simulink model "TX_TUNE_DIGITAL"  (R2024a)
settings: Solver=VariableStepAuto  StartTime=0.0  StopTime=1e-3  FixedStep=1e-9  RelTol=1e-3
values from neighbouring files (symbols this model uses):
  cnt_n_bits = 9    [TX_PM_MODEL_Setup.m]
  Cs = 12.5e-12    (= 1.25e-11)    [Oscillator_Setup.m]
  deltaVOSC = 0.5    [Oscillator_Setup.m]
  I0 = 100e-6    (= 0.0001)    [Oscillator_Setup.m]
  R = 0.2    [TX_PM_MODEL_Setup.m]
  Rf = 1e9    (= 1000000000)    [Oscillator_Setup.m]
  VDD = 5    [Oscillator_Setup.m]    (also in TX_PM_MODEL_Setup.m = 10)
  Vh = VDD - deltaVOSC    (= 4.5)    [Oscillator_Setup.m]
  Vl = deltaVOSC    (= 0.5)    [Oscillator_Setup.m]
undefined symbols (not defined in the file or in its folder): VDD_DRIVE
libraries: fl_lib x12, nesl_utility x7, MyLib x3, dspsigops x3, ee_lib x1, spsTriangleGeneratorLib x1
settings Model: Creator=cian.odonnell  LastModifiedBy=ciano
settings SolverCC: EnableFixedStepZeroCrossing=on

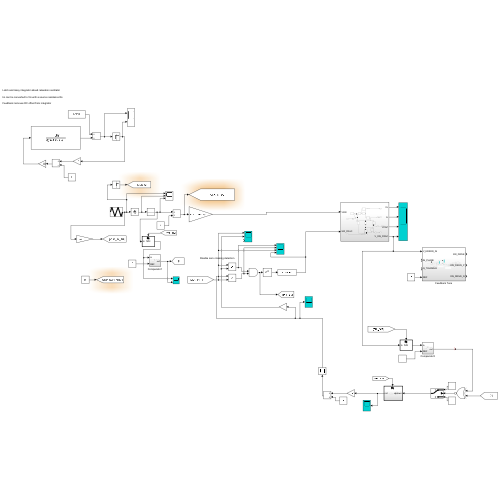
[thumbnail: Simulink's stored preview of the top-level diagram]
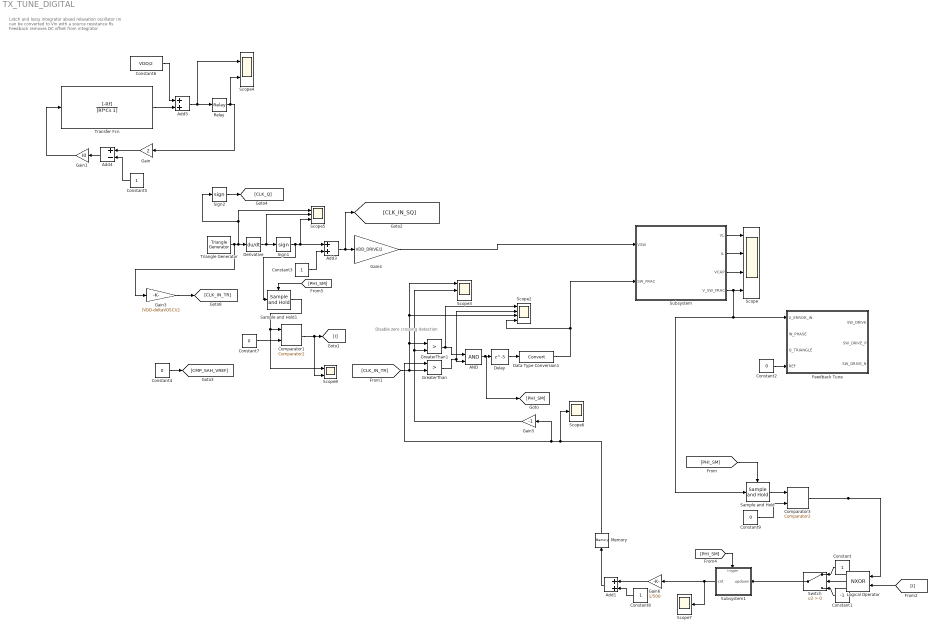
== system TX_TUNE_DIGITAL ==
  note: Latch and lossy integrator absed relaxation oscillator
      |
      | Iin can be converted to Vin with a source resistance Rs
      |
      | Feedback removes DC offset from integrator
  note: Disable zero crossing detection
  AND : Logic  IconShape=distinctive  AllPortsSameDT=off  OutDataTypeStr=boolean
  Add1 : Sum
  Add3 : Sum
  Add4 : Sum  Inputs=+-
  Add5 : Sum
  Comparator1 : MyLib/Comparator2  SystemSampleTime=-1  VariantActivationTime=update diagram  AllowFlexibleInterface=on  Latency=0  AutoFrameSizeCalculation=off
  Comparator3 : MyLib/Comparator2  SystemSampleTime=-1  VariantActivationTime=update diagram  AllowFlexibleInterface=on  Latency=0  AutoFrameSizeCalculation=off
  Constant{,3,5,8} (4 alike) : Constant
  Constant1 : Constant  Value=-1
  Constant{2,4,7,9} (4 alike) : Constant  Value=0
  Constant6 : Constant  Value=VDD/2
  Data Type Conversion1 : DataTypeConversion  SaturateOnIntegerOverflow=off  RndMeth=Floor
  Delay : Delay  DelayLength=5  SampleTime=1e-9
  Derivative : Derivative
  Feedback Tune : Subsystem
  Gain : Gain  Gain=2
  Gain1 : Gain  Gain=I0
  Gain3 : Gain  Gain=(VDD-deltaVOSC)/2
  Gain4 : Gain  Gain=VDD_DRIVE/2
  Gain5 : Gain  Gain=-1
  Gain6 : Gain  Gain=1/500
  GreaterThan : RelationalOperator  Operator=>  OutDataTypeStr=boolean  ZeroCross=off  RndMeth=Simplest  InputSameDT=off
  GreaterThan1 : RelationalOperator  Operator=>  OutDataTypeStr=boolean  ZeroCross=off  RndMeth=Simplest  InputSameDT=off
  Logical Operator : Logic  Operator=NXOR  IconShape=distinctive  AllPortsSameDT=off  OutDataTypeStr=boolean
  Memory : Memory
  Relay : Relay  OnSwitchValue=Vh  OffSwitchValue=Vl
  Sample and Hold : dspsigops/Sample and Hold  trig=Either edge  initCond=0  latchinput=off
  Sample and Hold1 : dspsigops/Sample and Hold  trig=Either edge  initCond=0  latchinput=off
  Scope : Scope  NumInputPorts=4
  Scope2 : Scope  NumInputPorts=4
  Scope3 : Scope  NumInputPorts=3
  Scope4 : Scope  NumInputPorts=2
  Scope5 : Scope  NumInputPorts=3
  Scope6 : Scope
  Scope7 : Scope
  Scope8 : Scope  NumInputPorts=2
  Sign1 : Signum
  Sign2 : Signum
  Subsystem : Subsystem
  Subsystem1 : Subsystem
  Switch : Switch  Criteria=u2 > Threshold  SaturateOnIntegerOverflow=off  InputSameDT=off
  Transfer Fcn : TransferFcn  Numerator=[-Rf]  Denominator=[Rf*Cs 1]
  Triangle Generator : spsTriangleGeneratorLib/Triangle Generator  Freq=fin  Phase=90  Ts=0
  wires:
  GreaterThan/1 -> Scope2/2, AND/2
  Add5/1 -> Scope4/1, Relay/1
  Transfer Fcn/1 -> Add5/2
  Gain1/1 -> Transfer Fcn/1
  Add4/1 -> Gain1/1
  Gain/1 -> Add4/1
  Constant5/1 -> Add4/2
  Constant6/1 -> Add5/1
  Relay/1 -> Gain/1, Scope4/2
  Gain3/1 -> [CLK_IN_TR]
  Triangle Generator/1 -> Sign2/1, Scope5/1, Derivative/1, Gain3/1
  Derivative/1 -> Sign1/1, Scope5/2
  Sign1/1 -> Sample and Hold1/1, Add3/1, Scope5/3
  Constant3/1 -> Add3/2
  Add3/1 -> [CLK_IN_SQ], Gain4/1
  [CLK_IN_TR] -> GreaterThan/2, GreaterThan1/1, Scope3/1, Scope2/3
  Gain5/1 -> GreaterThan1/2, Scope3/2
  GreaterThan1/1 -> Scope2/1, AND/1
  Data Type Conversion1/1 -> Scope2/4, Subsystem/2(SW_FRAC)
  AND/1 -> [PHI_SM], Delay/1
  Delay/1 -> Data Type Conversion1/1
  [I] -> Logical Operator/2
  Gain4/1 -> Subsystem/1(VSW)
  Subsystem/1(VL) -> Scope/1
  Subsystem/2(IL) -> Scope/2
  Subsystem/3(VCAP) -> Scope/3
  Comparator1/1 -> Scope8/2, [I]
  Constant4/1 -> [CMP_SAH_VREF]
  Constant7/1 -> Comparator1/2
  Sign2/1 -> [CLK_Q]
  Add1/1 -> Memory/1
  [PHI_SM] -> Subsystem1/Trigger
  Subsystem1/1(cnt) -> Gain6/1, Scope7/1
  Switch/1 -> Subsystem1/1(updown)
  Sample and Hold1/1 -> Comparator1/1, Scope8/1
  [PHI_SM] -> Sample and Hold1/Trigger
  Logical Operator/1 -> Switch/2
  Constant/1 -> Switch/1
  Constant1/1 -> Switch/3
  Gain6/1 -> Add1/1
  Constant8/1 -> Add1/2
  Memory/1 -> Scope6/1, GreaterThan/1, Gain5/1
  Constant2/1 -> Feedback Tune/4(REF)
  Comparator3/1 -> Logical Operator/1
  Sample and Hold/1 -> Comparator3/1
  Subsystem/4(V_SW_FRAC) -> Sample and Hold/1, Feedback Tune/1(V_ERROR_IN), Scope/4
  Constant9/1 -> Comparator3/2
  [PHI_SM] -> Sample and Hold/Trigger

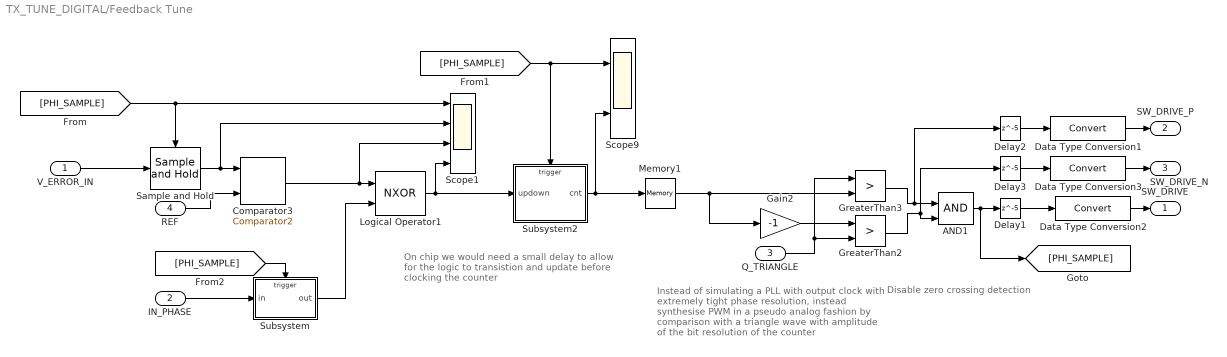
== system TX_TUNE_DIGITAL/Feedback Tune ==
  note: On chip we would need a small delay to allow for the logic to transistion and update before clocking the counter
  note: Disable zero crossing detection
  note: Instead of simulating a PLL with output clock with extremely tight phase resolution, instead synthesise PWM in a pseudo analog fashion by comparison with a triangle wave with amplitude of the bit resolution of the counter
  V_ERROR_IN : Inport
  IN_PHASE : Inport  Port=2
  Q_TRIANGLE : Inport  Port=3
  REF : Inport  Port=4
  AND1 : Logic  IconShape=distinctive  AllPortsSameDT=off  OutDataTypeStr=boolean
  Comparator3 : MyLib/Comparator2  SystemSampleTime=-1  VariantActivationTime=update diagram  AllowFlexibleInterface=on  Latency=0  AutoFrameSizeCalculation=off
  Data Type Conversion1 : DataTypeConversion  SaturateOnIntegerOverflow=off  RndMeth=Floor
  Data Type Conversion2 : DataTypeConversion  SaturateOnIntegerOverflow=off  RndMeth=Floor
  Data Type Conversion3 : DataTypeConversion  SaturateOnIntegerOverflow=off  RndMeth=Floor
  Delay1 : Delay  DelayLength=5  SampleTime=1e-9
  Delay2 : Delay  DelayLength=5  SampleTime=1e-9
  Delay3 : Delay  DelayLength=5  SampleTime=1e-9
  Gain2 : Gain  Gain=-1
  GreaterThan2 : RelationalOperator  Operator=>  OutDataTypeStr=boolean  ZeroCross=off  RndMeth=Simplest  InputSameDT=off
  GreaterThan3 : RelationalOperator  Operator=>  OutDataTypeStr=boolean  ZeroCross=off  RndMeth=Simplest  InputSameDT=off
  Logical Operator1 : Logic  Operator=NXOR  IconShape=distinctive  AllPortsSameDT=off  OutDataTypeStr=boolean
  Memory1 : Memory
  Sample and Hold : dspsigops/Sample and Hold  trig=Either edge  initCond=0  latchinput=off
  Scope1 : Scope  NumInputPorts=4
  Scope9 : Scope  NumInputPorts=2
  Subsystem : Subsystem
  Subsystem2 : Subsystem
  SW_DRIVE : Outport
  SW_DRIVE_P : Outport  Port=2
  SW_DRIVE_N : Outport  Port=3
  wires:
  [PHI_SAMPLE] -> Sample and Hold/Trigger, Scope1/1
  Gain2/1 -> GreaterThan2/1
  Subsystem2/1(cnt) -> Memory1/1, Scope9/2
  Delay1/1 -> Data Type Conversion2/1
  Sample and Hold/1 -> Scope1/2, Comparator3/1
  Logical Operator1/1 -> Subsystem2/1(updown), Scope1/4
  Comparator3/1 -> Scope1/3, Logical Operator1/1
  Memory1/1 -> Gain2/1, GreaterThan3/2
  Q_TRIANGLE/1 -> GreaterThan2/2, GreaterThan3/1
  [PHI_SAMPLE] -> Subsystem2/Trigger, Scope9/1
  GreaterThan3/1 -> Delay2/1, AND1/1
  AND1/1 -> [PHI_SAMPLE], Delay1/1
  GreaterThan2/1 -> Delay3/1, AND1/2
  Data Type Conversion2/1 -> SW_DRIVE/1
  V_ERROR_IN/1 -> Sample and Hold/1
  REF/1 -> Comparator3/2
  IN_PHASE/1 -> Subsystem/1(in)
  Subsystem/1(out) -> Logical Operator1/2
  [PHI_SAMPLE] -> Subsystem/Trigger
  Delay2/1 -> Data Type Conversion1/1
  Delay3/1 -> Data Type Conversion3/1
  Data Type Conversion1/1 -> SW_DRIVE_P/1
  Data Type Conversion3/1 -> SW_DRIVE_N/1

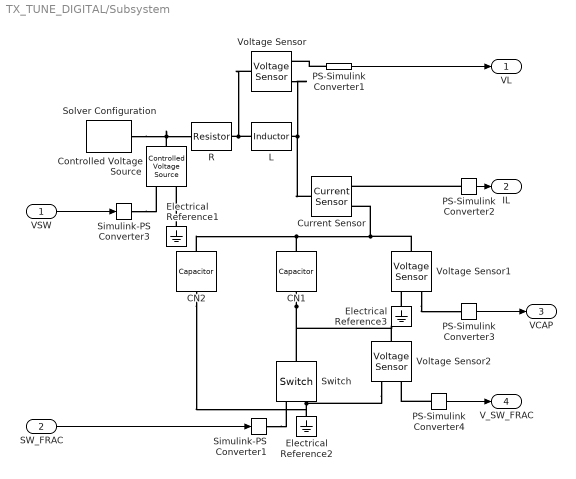
== system TX_TUNE_DIGITAL/Subsystem ==
  VSW : Inport
  SW_FRAC : Inport  Port=2
  CN1 : fl_lib/Electrical/Electrical Elements/Capacitor  c=3e-9 F  r=1e-6 Ohm  g=0 1/Ohm  i_specify=off  i_priority=None  i=0 A  i_nominal_specify=off  i_nominal_value=1  i_nominal_unit=A  v_specify=off  v_priority=None  v=0 V  v_nominal_specify=off  v_nominal_value=1  v_nominal_unit=V  vc_specify=off  vc_priority=High  vc=0 V  vc_nominal_specify=off  vc_nominal_value=1  vc_nominal_unit=V
  CN2 : fl_lib/Electrical/Electrical Elements/Capacitor  c=3e-9 F  r=1e-6 Ohm  g=0 1/Ohm  i_specify=off  i_priority=None  i=0 A  i_nominal_specify=off  i_nominal_value=1  i_nominal_unit=A  v_specify=off  v_priority=None  v=0 V  v_nominal_specify=off  v_nominal_value=1  v_nominal_unit=V  vc_specify=off  vc_priority=High  vc=0 V  vc_nominal_specify=off  vc_nominal_value=1  vc_nominal_unit=V
  Controlled Voltage Source : fl_lib/Electrical/Electrical Sources/Controlled Voltage Source
  Current Sensor : fl_lib/Electrical/Electrical Sensors/Current Sensor
  Electrical Reference1 : fl_lib/Electrical/Electrical Elements/Electrical Reference
  Electrical Reference2 : fl_lib/Electrical/Electrical Elements/Electrical Reference
  Electrical Reference3 : fl_lib/Electrical/Electrical Elements/Electrical Reference
  L : ee_lib/Passive/Inductor  l=L H  enable_L_tol=ee.enum.toleranceApplication.none  L_tol=20  tol_distribution=ee.enum.toleranceDistribution.uniform  nSigma=4  r=0 Ohm  g=1e-9 1/Ohm  enable_operating_limits=ee.enum.enable.no  operating_limit_action=ee.enum.passive.reportOpLim.warn  max_working_current=1 A  power_rating=1 W  enable_faults=ee.enum.enable.no  fault_action=simscape.enum.assert.action.none  lambdaPercent=50  k_faulted=0.9999  turnsShort=ee.enum.passive.inductor.turnsShortOption.no  openCct=ee.enum.enable.no  groundShort=ee.enum.passive.inductor.groundShortOption.no  groundShortG=0 1/Ohm  tau_fault=1e-3 s  fault_trigger=ee.enum.faults.faultTrigger.temporal  t_fault=1 s  max_permissible_voltage=100 V  n_fail_on_voltage=1  max_permissible_current=1 A  t_fail_on_current=1 s  i_L_specify=off  i_L_priority=High  i_L=0 A  i_L_nominal_specify=off  i_L_nominal_value=1  i_L_nominal_unit=A  faulted_specify=off  faulted_priority=None  faulted=0
  PS-Simulink Converter{1..4} (4 alike) : nesl_utility/PS-Simulink Converter  PhysicalDomain=network_engine_domain  SubClassName=ps_output  LeftPortType=input  RightPortType=output  PseudoPeriodic=off  Frequencies=[]  VectorFormat=inherit  Unit=inherit  AffineConversion=off
  R : fl_lib/Electrical/Electrical Elements/Resistor  R=R Ohm  i_specify=off  i_priority=None  i=0 A  i_nominal_specify=off  i_nominal_value=1  i_nominal_unit=A  v_specify=off  v_priority=None  v=0 V  v_nominal_specify=off  v_nominal_value=1  v_nominal_unit=V
  Simulink-PS Converter1 : nesl_utility/Simulink-PS Converter  PhysicalDomain=network_engine_domain  SubClassName=ps_input  LeftPortType=input  RightPortType=output  PseudoPeriodic=off  Frequencies=[]  NoiseDistribution=none  NoiseParameters=[]  Unit=1  AffineConversion=off  FilteringAndDerivatives=provide  SimscapeFilterOrder=1  InputFilterTimeConstant=0.001  UdotUserProvided=0
  Simulink-PS Converter3 : nesl_utility/Simulink-PS Converter  PhysicalDomain=network_engine_domain  SubClassName=ps_input  LeftPortType=input  RightPortType=output  PseudoPeriodic=off  Frequencies=[]  NoiseDistribution=none  NoiseParameters=[]  Unit=1  AffineConversion=off  FilteringAndDerivatives=provide  SimscapeFilterOrder=1  InputFilterTimeConstant=0.001  UdotUserProvided=0
  Solver Configuration : nesl_utility/Solver Configuration  PhysicalDomain=network_engine_domain  SubClassName=solver  LeftPortType=input  RightPortType=generic  Tones=[]  Harmonics=[]  SimulateNoise=off  Profile=off  UseLocalSampling=off  EnableSwitchedLinearOptims=on  FrequencyDomain=off  UseCCode=off  RelTol=0.001  AbsTol=0.001  MinStep=1e-09  ToWorkspace=off  RevertToSquareIcSolve=off  NumHomotopyIterations=100  PhasorMode=off  PhasorModeNumHarmonics=1  ConsistencySolver=NEWTON_XTOL_AFTER_FTOL  IndexReductionMethod=DerivativeReplacement  DoDC=off  ResidualTolerance=1e-09  ConsistencyTolSource=GLOBAL  ConsistencyAbsTol=0.001  ConsistencyRelTol=0.001  ConsistencyTolFactor=0.001  UseLocalSolver=off  LocalSolverChoice=NE_BACKWARD_EULER_ADVANCER  ResolveIndetEquations=on  FunctionEvalNumThread=1  LocalSolverSampleTime=0.001  DoFixedCost=off  MaxNonlinIter=3  MaxModeIter=2  ComputeImpulses=off  ImpulseIterations=2  LinearAlgebra=auto  LinearAlgebraNumThread=0  EquationFormulation=NE_TIME_EF  DelaysMemoryBudget=1024  AutomaticFiltering=on  FilteringTimeConstant=0.001  PartitionStorageMethod=AS_NEEDED  PartitionMemoryBudget=1024  PartitionMethod=ROBUST  MultibodyUseLocalSolver=off  MultibodyLocalSolverChoice=ODE1  MultibodyLocalSolverSampleTime=0.001
  Switch : fl_lib/Electrical/Electrical Elements/Switch  R_closed=0.01 Ohm  G_open=1e-8 1/Ohm  Threshold=0.5  i_specify=off  i_priority=None  i=0 A  i_nominal_specify=off  i_nominal_value=1  i_nominal_unit=A  v_specify=off  v_priority=None  v=0 V  v_nominal_specify=off  v_nominal_value=1  v_nominal_unit=V
  Voltage Sensor : fl_lib/Electrical/Electrical Sensors/Voltage Sensor
  Voltage Sensor1 : fl_lib/Electrical/Electrical Sensors/Voltage Sensor
  Voltage Sensor2 : fl_lib/Electrical/Electrical Sensors/Voltage Sensor
  VL : Outport
  IL : Outport  Port=2
  VCAP : Outport  Port=3
  V_SW_FRAC : Outport  Port=4
  wires:
  PS-Simulink Converter3/1 -> VCAP/1
  SW_FRAC/1 -> Simulink-PS Converter1/1
  PS-Simulink Converter2/1 -> IL/1
  PS-Simulink Converter4/1 -> V_SW_FRAC/1
  VSW/1 -> Simulink-PS Converter3/1
  PS-Simulink Converter1/1 -> VL/1
  connections:
  Current Sensor/LConn1 -- Voltage Sensor/RConn2 -- L/RConn1
  Electrical Reference1/LConn1 -- Controlled Voltage Source/RConn2
  Voltage Sensor1/RConn1 -- PS-Simulink Converter3/LConn1
  Electrical Reference3/LConn1 -- Voltage Sensor1/RConn2
  CN1/RConn1 -- Voltage Sensor2/LConn1 -- Switch/LConn1
  Simulink-PS Converter3/RConn1 -- Controlled Voltage Source/RConn1
  CN1/LConn1 -- Voltage Sensor1/LConn1 -- Current Sensor/RConn2 -- CN2/LConn1
  PS-Simulink Converter2/LConn1 -- Current Sensor/RConn1
  PS-Simulink Converter1/LConn1 -- Voltage Sensor/RConn1
  Electrical Reference2/LConn1 -- CN2/RConn1 -- Switch/RConn2 -- Voltage Sensor2/RConn2
  Simulink-PS Converter1/RConn1 -- Switch/RConn1
  PS-Simulink Converter4/LConn1 -- Voltage Sensor2/RConn1
  L/LConn1 -- Voltage Sensor/LConn1 -- R/RConn1
  Controlled Voltage Source/LConn1 -- R/LConn1 -- Solver Configuration/RConn1

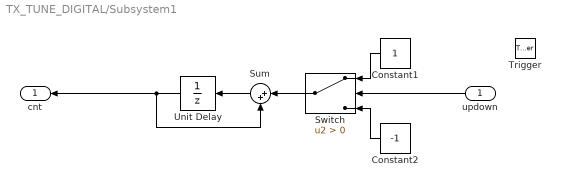
== system TX_TUNE_DIGITAL/Subsystem1 ==
  updown : Inport
  Trigger : TriggerPort  TriggerType=either  VariantControl=(inherit)  PortDimensions=1
  Constant1 : Constant
  Constant2 : Constant  Value=-1
  Sum : Sum  Inputs=|++
  Switch : Switch  Criteria=u2 > Threshold  SaturateOnIntegerOverflow=off  InputSameDT=off
  Unit Delay : UnitDelay  SampleTime=-1  HasFrameUpgradeWarning=on
  cnt : Outport
  wires:
  Switch/1 -> Sum/1
  Constant2/1 -> Switch/3
  Sum/1 -> Unit Delay/1
  updown/1 -> Switch/2
  Unit Delay/1 -> cnt/1, Sum/2
  Constant1/1 -> Switch/1

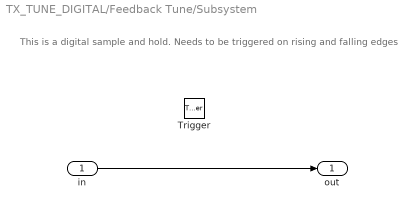
== system TX_TUNE_DIGITAL/Feedback Tune/Subsystem ==
  note: This is a digital sample and hold. Needs to be triggered on rising and falling edges
  in : Inport
  Trigger : TriggerPort  TriggerType=either  VariantControl=(inherit)  PortDimensions=1
  out : Outport
  wires:
  in/1 -> out/1

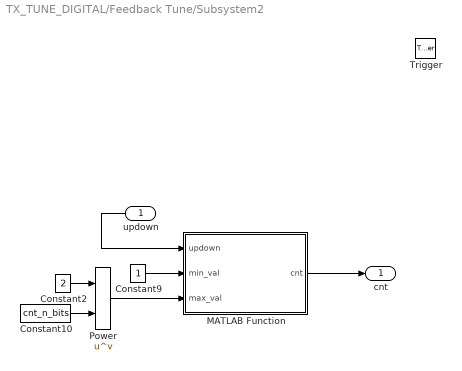
== system TX_TUNE_DIGITAL/Feedback Tune/Subsystem2 ==
  updown : Inport
  Trigger : TriggerPort  TriggerType=either  VariantControl=(inherit)  PortDimensions=1
  Constant10 : Constant  Value=cnt_n_bits
  Constant2 : Constant  Value=2
  Constant9 : Constant
  MATLAB Function : MATLAB Function  TreatAsAtomicUnit=on
  Power : Math  Operator=pow
  cnt : Outport
  wires:
  Constant10/1 -> Power/2
  Constant2/1 -> Power/1
  Constant9/1 -> MATLAB Function/2(min_val)
  Power/1 -> MATLAB Function/3(max_val)
  MATLAB Function/1(cnt) -> cnt/1
  updown/1 -> MATLAB Function/1(updown)

== matlab function TX_TUNE_DIGITAL/Feedback Tune/Subsystem2/MATLAB Function ==
  data: updown input; cnt output; min_val input; max_val input
function cnt = updown_cnt(updown, min_val, max_val)
    % updown: 1 = UP, 0 = DOWN
    
    persistent current_count;

    % Initialize at min_val on the very first step
    if isempty(current_count)
        current_count = min_val;
    end

    % Logic: Convert Boolean updown (0 or 1) to -1 or +1
    if updown == 1
        current_count = current_count + 1;
    else
        current_count = current_count - 1;
    end

    % Enforce Limits (Saturation)
    if current_count > max_val
        current_count = max_val;
    elseif current_count < min_val
        current_count = min_val;
    end

    % Assign internal state to the output variable 'cnt'
    cnt = current_count;
end
